simulink model "sb_systeme"  (R2016a)
settings: Solver=VariableStepAuto  StartTime=0.0  StopTime=10.0  RelTol=1e-3
undefined symbols (not defined in the file): g, Js, LA, LB, LC, ms, mtot, RA, RB, RC, Va, Vb, Vc, XA, XB, XC, YA, YB, YC
settings Model: Creator=whij1602  LastModifiedBy=whij1602

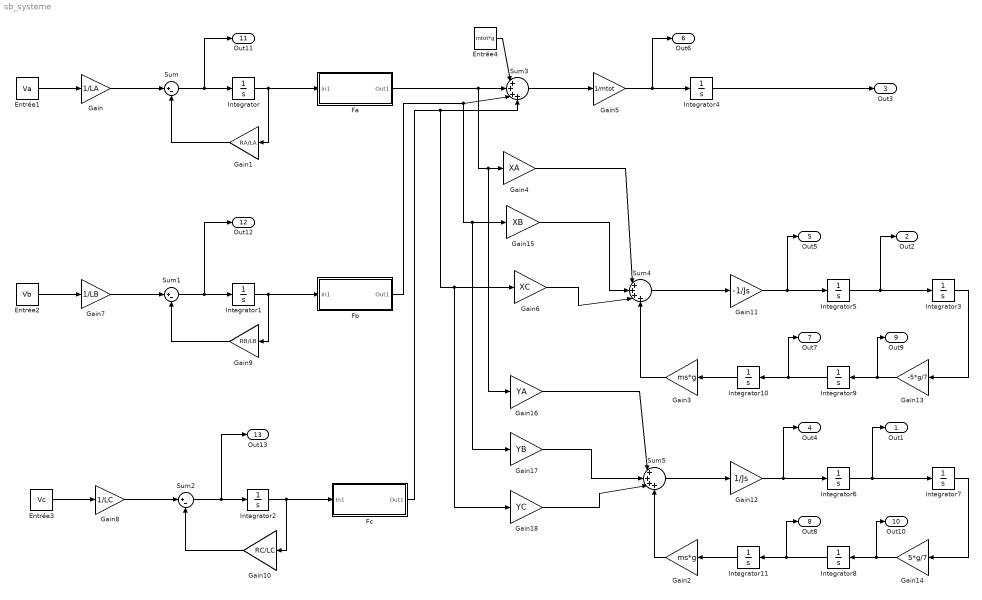
== system sb_systeme ==
  Entrée1 : Constant  Value=Va
  Entrée2 : Constant  Value=Vb
  Entrée3 : Constant  Value=Vc
  Entrée4 : Constant  Value=mtot*g
  Fa : Subsystem
  Fb : Subsystem
  Fc : Subsystem
  Gain : Gain  Gain=1/LA
  Gain1 : Gain  Gain=RA/LA
  Gain10 : Gain  Gain=RC/LC
  Gain11 : Gain  Gain=-1/Js
  Gain12 : Gain  Gain=1/Js
  Gain13 : Gain  Gain=-5*g/7
  Gain14 : Gain  Gain=5*g/7
  Gain15 : Gain  Gain=XB
  Gain16 : Gain  Gain=YA
  Gain17 : Gain  Gain=YB
  Gain18 : Gain  Gain=YC
  Gain2 : Gain  Gain=ms*g
  Gain3 : Gain  Gain=ms*g
  Gain4 : Gain  Gain=XA
  Gain5 : Gain  Gain=1/mtot
  Gain6 : Gain  Gain=XC
  Gain7 : Gain  Gain=1/LB
  Gain8 : Gain  Gain=1/LC
  Gain9 : Gain  Gain=RB/LB
  Integrator{,1..11} (12 alike) : Integrator
  Sum : Sum  Inputs=|+-
  Sum1 : Sum  Inputs=|+-
  Sum2 : Sum  Inputs=|+-
  Sum3 : Sum  Inputs=|++++
  Sum4 : Sum  Inputs=|++++
  Sum5 : Sum  Inputs=|++++
  Out1 : Outport
  Out2 : Outport  Port=2
  Out3 : Outport  Port=3
  Out4 : Outport  Port=4
  Out5 : Outport  Port=5
  Out6 : Outport  Port=6
  Out7 : Outport  Port=7
  Out8 : Outport  Port=8
  Out9 : Outport  Port=9
  Out10 : Outport  Port=10
  Out11 : Outport  Port=11
  Out12 : Outport  Port=12
  Out13 : Outport  Port=13
  wires:
  Entrée3/1 -> Gain8/1
  Gain8/1 -> Sum2/1
  Sum2/1 -> Out13/1, Integrator2/1
  Entrée2/1 -> Gain7/1
  Gain7/1 -> Sum1/1
  Sum1/1 -> Out12/1, Integrator1/1
  Entrée1/1 -> Gain/1
  Gain/1 -> Sum/1
  Sum/1 -> Out11/1, Integrator/1
  Integrator/1 -> Gain1/1, Fa/1(In1)
  Gain1/1 -> Sum/2
  Integrator1/1 -> Fb/1(In1), Gain9/1
  Gain9/1 -> Sum1/2
  Integrator2/1 -> Fc/1(In1), Gain10/1
  Gain10/1 -> Sum2/2
  Entrée4/1 -> Sum3/1
  Fa/1(Out1) -> Gain16/1, Gain4/1, Sum3/2
  Sum3/1 -> Gain5/1
  Gain5/1 -> Out6/1, Integrator4/1
  Sum5/1 -> Gain12/1
  Sum4/1 -> Gain11/1
  Gain11/1 -> Out5/1, Integrator5/1
  Gain12/1 -> Out4/1, Integrator6/1
  Integrator5/1 -> Out2/1, Integrator3/1
  Integrator6/1 -> Out1/1, Integrator7/1
  Integrator7/1 -> Gain14/1
  Integrator3/1 -> Gain13/1
  Gain14/1 -> Out10/1, Integrator8/1
  Gain13/1 -> Out9/1, Integrator9/1
  Integrator9/1 -> Out7/1, Integrator10/1
  Integrator8/1 -> Out8/1, Integrator11/1
  Integrator11/1 -> Gain2/1
  Gain2/1 -> Sum5/4
  Integrator10/1 -> Gain3/1
  Gain3/1 -> Sum4/4
  Integrator4/1 -> Out3/1
  Fb/1(Out1) -> Gain17/1, Gain15/1, Sum3/3
  Fc/1(Out1) -> Gain18/1, Gain6/1, Sum3/4
  Gain4/1 -> Sum4/1
  Gain15/1 -> Sum4/2
  Gain6/1 -> Sum4/3
  Gain16/1 -> Sum5/1
  Gain17/1 -> Sum5/2
  Gain18/1 -> Sum5/3

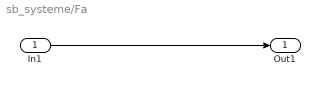
== system sb_systeme/Fa ==
  In1 : Inport
  Out1 : Outport
  wires:
  In1/1 -> Out1/1

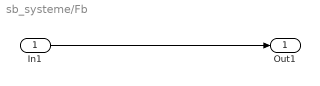
== system sb_systeme/Fb ==
  In1 : Inport
  Out1 : Outport
  wires:
  In1/1 -> Out1/1

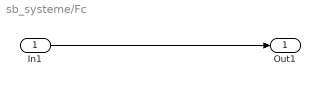
== system sb_systeme/Fc ==
  In1 : Inport
  Out1 : Outport
  wires:
  In1/1 -> Out1/1
